simulink model "pidCascade_struc2_Tuner"  (R2015b)
settings: Solver=ode15s  StartTime=0.0  StopTime=20*3600  FixedStep=10  MaxStep=20  MinStep=10  RelTol=1e-8  AbsTol=1e-8
settings Model: Creator=Administrator  LastModifiedBy=Administrator
settings SolverCC: InitialStep=12
settings DataIOCC: SaveFormat=Array  SignalLogging=off
settings DebuggingCC: UnderspecifiedInitializationDetection=Classic  MergeDetectMultiDrivingBlocksExec=none  SolverPrmCheckMsg=warning  StateNameClashWarn=warning
settings HardwareCC: ProdBitPerPointer=32  ProdLargestAtomicFloat=None  ProdIntDivRoundTo=Undefined  ProdEndianess=Unspecified  ProdWordSize=32  ProdHWDeviceType=32-bit Generic
settings GRTTargetCC: GeneratePreprocessorConditionals=Disable all
settings ConfigComp: CovModelRefEnable=Off

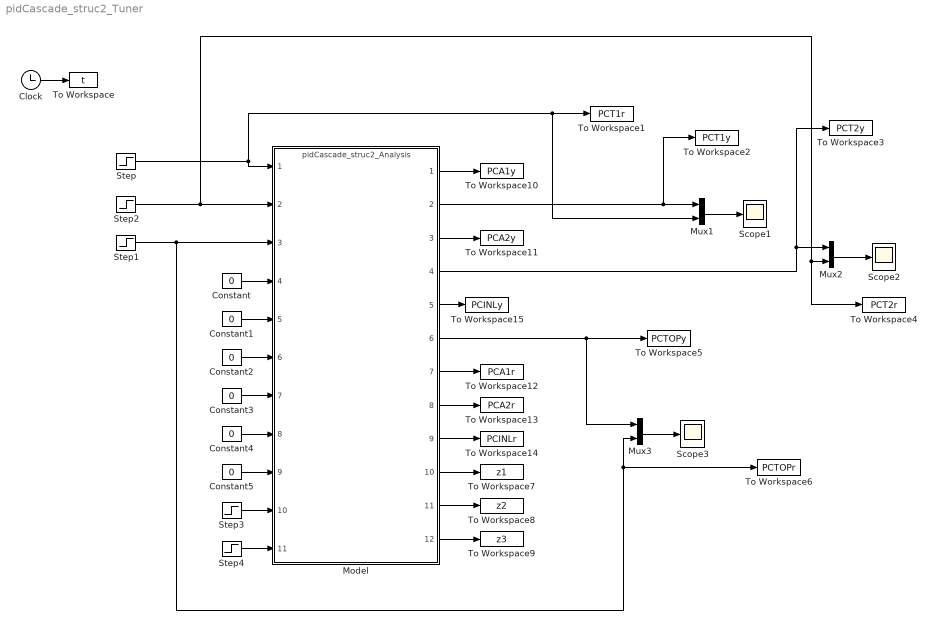
== system pidCascade_struc2_Tuner ==
  Clock : Clock
  Constant{,1..5} (6 alike) : Constant  Value=0
  Model : ModelReference  ModelNameDialog=pidCascade_struc2_Analysis.slx  SimulationMode=Normal  ModelReferenceVersion=1.95  CopyOfModelName=pidCascade_struc2_Analysis.slx
  Mux1 : Mux  Inputs=2
  Mux2 : Mux  Inputs=2
  Mux3 : Mux  Inputs=2
  Scope1 : Scope
  Scope2 : Scope
  Scope3 : Scope
  Step : Step  Time=8*3600  After=-2e4  SampleTime=0
  Step1 : Step  Time=16*3600  After=-1e4  SampleTime=0
  Step2 : Step  Time=12*3600  After=-2e4  SampleTime=0
  Step3 : Step  Time=1*3600  After=0.05  SampleTime=0
  Step4 : Step  Time=4*3600  After=0.05  SampleTime=0
  To Workspace : ToWorkspace  VariableName=t  SampleTime=-1
  To Workspace1 : ToWorkspace  VariableName=PCT1r  SampleTime=-1
  To Workspace10 : ToWorkspace  VariableName=PCA1y  SampleTime=-1
  To Workspace11 : ToWorkspace  VariableName=PCA2y  SampleTime=-1
  To Workspace12 : ToWorkspace  VariableName=PCA1r  SampleTime=-1
  To Workspace13 : ToWorkspace  VariableName=PCA2r  SampleTime=-1
  To Workspace14 : ToWorkspace  VariableName=PCINLr  SampleTime=-1
  To Workspace15 : ToWorkspace  VariableName=PCINLy  SampleTime=-1
  To Workspace2 : ToWorkspace  VariableName=PCT1y  SampleTime=-1
  To Workspace3 : ToWorkspace  VariableName=PCT2y  SampleTime=-1
  To Workspace4 : ToWorkspace  VariableName=PCT2r  SampleTime=-1
  To Workspace5 : ToWorkspace  VariableName=PCTOPy  SampleTime=-1
  To Workspace6 : ToWorkspace  VariableName=PCTOPr  SampleTime=-1
  To Workspace7 : ToWorkspace  VariableName=z1  SampleTime=-1
  To Workspace8 : ToWorkspace  VariableName=z2  SampleTime=-1
  To Workspace9 : ToWorkspace  VariableName=z3  SampleTime=-1
  wires:
  Model/2 -> To Workspace2/1, Mux1/1
  Model/4 -> To Workspace3/1, Mux2/1
  Step/1 -> To Workspace1/1, Mux1/2, Model/1
  Step2/1 -> To Workspace4/1, Mux2/2, Model/2
  Step1/1 -> To Workspace6/1, Mux3/2, Model/3
  Mux1/1 -> Scope1/1
  Mux2/1 -> Scope2/1
  Clock/1 -> To Workspace/1
  Mux3/1 -> Scope3/1
  Constant/1 -> Model/4
  Constant1/1 -> Model/5
  Constant2/1 -> Model/6
  Constant3/1 -> Model/7
  Model/1 -> To Workspace10/1
  Model/3 -> To Workspace11/1
  Constant4/1 -> Model/8
  Constant5/1 -> Model/9
  Model/12 -> To Workspace9/1
  Model/11 -> To Workspace8/1
  Model/10 -> To Workspace7/1
  Model/8 -> To Workspace13/1
  Model/7 -> To Workspace12/1
  Model/6 -> Mux3/1, To Workspace5/1
  Model/9 -> To Workspace14/1
  Model/5 -> To Workspace15/1
  Step3/1 -> Model/10
  Step4/1 -> Model/11
